simulink model "InverseKinematics"  (R2023b)
settings: Solver=VariableStepAuto  StartTime=0.0  StopTime=30  RelTol=1e-3
undefined symbols (not defined in the file or in its folder): Levenberg, Marquardt, num_points
libraries: simulink x3, robotcorelib x1, robotmaniplib x1
settings Model: Creator=Camo  LastModifiedBy=Camo

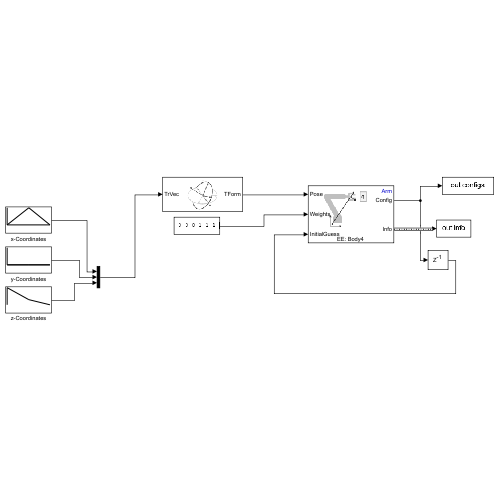
[thumbnail: Simulink's stored preview of the top-level diagram]
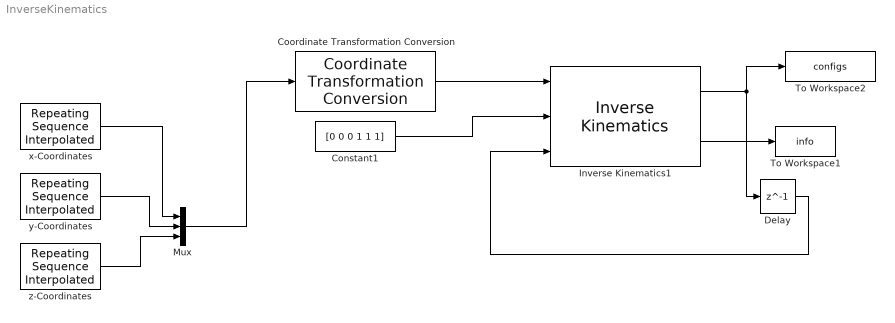
== system InverseKinematics ==
  Constant1 : Constant  Value=[0 0 0 1 1 1]
  Coordinate Transformation Conversion : robotcorelib/Coordinate Transformation Conversion  InputRepresentation=Translation Vector  InputEulerSequence=ZYX  ShowTrVecInputPort=on  OutputRepresentation=Homogeneous Transformation  OutputEulerSequence=ZYX  ShowTrVecOutputPort=on  SimulateUsing=Interpreted execution
  Delay : Delay  DelayLength=1  InitialCondition=zeros(3,1)
  Inverse Kinematics1 : robotmaniplib/Inverse Kinematics  RigidBodyTree=Arm  EndEffector=Body4  ShowInfo=on  SolverName=Levenberg-Marquardt  EnforceJointLimits=on  MaxIterations=1500  MaxTime=10  GradientTolerance=1e-7  SolutionTolerance=1e-6  StepTolerance=1e-14  ErrorChangeTolerance=1e-12  UseErrorDamping=on  DampingBias=0.0025  SimulateUsing=Interpreted execution
  Mux : Mux  Inputs=3
  To Workspace1 : ToWorkspace  VariableName=info  SaveFormat=Timeseries  SampleTime=-1
  To Workspace2 : ToWorkspace  VariableName=configs  SaveFormat=Timeseries  SampleTime=-1
  "x-Coordinates " : simulink/Sources/Repeating Sequence Interpolated  OutValues=x  TimeValues=linspace(0,15,num_points)  LookUpMeth=Interpolation-Use End Values  tsamp=0.01  OutMin=[]  OutMax=[]  OutDataTypeStr=double  OutputDataTypeScalingMode=double  OutDataType=fixdt(0,8)  OutScaling=2^-10
  y-Coordinates : simulink/Sources/Repeating Sequence Interpolated  OutValues=y  TimeValues=linspace(0,15,num_points)  LookUpMeth=Interpolation-Use End Values  tsamp=0.01  OutMin=[]  OutMax=[]  OutDataTypeStr=double  OutputDataTypeScalingMode=double  OutDataType=fixdt(0,8)  OutScaling=2^-10
  z-Coordinates : simulink/Sources/Repeating Sequence Interpolated  OutValues=z  TimeValues=linspace(0,15,num_points)  LookUpMeth=Interpolation-Use End Values  tsamp=0.01  OutMin=[]  OutMax=[]  OutDataTypeStr=double  OutputDataTypeScalingMode=double  OutDataType=fixdt(0,8)  OutScaling=2^-10
  wires:
  Inverse Kinematics1/2 -> To Workspace1/1
  Inverse Kinematics1/1 -> To Workspace2/1, Delay/1
  Delay/1 -> Inverse Kinematics1/3
  Mux/1 -> Coordinate Transformation Conversion/1
  Constant1/1 -> Inverse Kinematics1/2
  Coordinate Transformation Conversion/1 -> Inverse Kinematics1/1
  z-Coordinates/1 -> Mux/3
  y-Coordinates/1 -> Mux/2
  "x-Coordinates "/1 -> Mux/1
